simulink model "HeartCode"  (R2020a)
settings: Solver=FixedStepAuto  StartTime=0.0  StopTime=10.0  FixedStep=1e-3  RelTol=1e-3  EnableMultiTasking=on
undefined symbols (not defined in the file): A0, A1, D0, D1, D10, D11, D12, D13, D2, D3, D4, D5, D6, D7, D8, D9, PTA0, PTA1, PTA2, PTB2, PTB23, PTB3, PTB9, PTC16, PTC17, PTC2, PTC3, PTC4, PTD0, PTD1, PTD2, PTD3
libraries: frdmk64flib x21, etargetslib x10
settings Model: ExtModeTrigDuration=5  Creator=user  LastModifiedBy=user
settings OptimizationCC: EnhancedBackFolding=on  PassReuseOutputArgsAs=Individual arguments  ZeroExternalMemoryAtStartup=off  ZeroInternalMemoryAtStartup=off  MaxStackSize=64  OptimizeBlockOrder=speed  DifferentSizesBufferReuse=on  OptimizationCustomize=off  EfficientTunableParamExpr=on
settings DebuggingCC: ParameterTunabilityLossMsg=error
settings HardwareCC: ProdBitPerPointer=32  ProdBitPerSizeT=32  ProdBitPerPtrDiffT=32  ProdLargestAtomicInteger=Long  ProdLargestAtomicFloat=Double  ProdWordSize=32  ProdHWDeviceType=ARM Compatible->ARM Cortex
settings SFSimCC: MATLABDynamicMemAlloc=off
settings RTWCC: SystemTargetFile=ert.tlc  HardwareBoard=NXP FRDM-K64F  TemplateMakefile=ert_default_tmf  Toolchain=GNU Tools for ARM Embedded Processors
settings CodeAppCC: ForceParamTrailComments=on  IgnoreCustomStorageClasses=off  OperatorAnnotations=on  SimulinkDataObjDesc=on  SFDataObjDesc=on  InsertBlockDesc=on

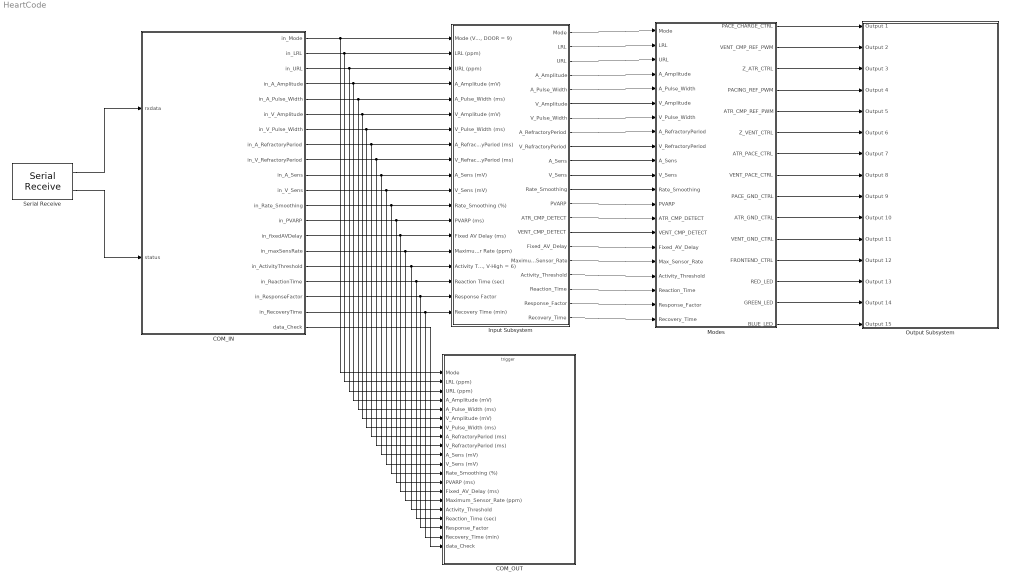
== system HeartCode ==
  COM_IN : Stateflow chart  TreatAsAtomicUnit=on
  COM_OUT : Subsystem  TreatAsAtomicUnit=on
  Input Subsystem : Subsystem
  Modes : Stateflow chart  TreatAsAtomicUnit=on
  Output Subsystem : Subsystem
  Serial Receive : frdmk64flib/Serial Receive  SCIModule=0  Baudrate=uint32(9600)  Parity=None  StopBits=1  HardwareFlowControl=None  ByteOrder=LittleEndian  DataType=uint8  DataLength=33  BlockingMode=off  OutputStatus=on  SampleTime=-1
  wires:
  Modes/1(PACE_CHARGE_CTRL) -> Output Subsystem/1(Output 1)
  Modes/2(VENT_CMP_REF_PWM) -> Output Subsystem/2(Output 2)
  Modes/3(Z_ATR_CTRL) -> Output Subsystem/3(Output 3)
  Modes/4(PACING_REF_PWM) -> Output Subsystem/4(Output 4)
  Modes/5(ATR_CMP_REF_PWM) -> Output Subsystem/5(Output 5)
  Modes/6(Z_VENT_CTRL) -> Output Subsystem/6(Output 6)
  Modes/7(ATR_PACE_CTRL) -> Output Subsystem/7(Output 7)
  Modes/8(VENT_PACE_CTRL) -> Output Subsystem/8(Output 8)
  Modes/9(PACE_GND_CTRL) -> Output Subsystem/9(Output 9)
  Modes/10(ATR_GND_CTRL) -> Output Subsystem/10(Output 10)
  Modes/11(VENT_GND_CTRL) -> Output Subsystem/11(Output 11)
  Modes/12(FRONTEND_CTRL) -> Output Subsystem/12(Output 12)
  Modes/13(RED_LED) -> Output Subsystem/13(Output 13)
  Modes/14(GREEN_LED) -> Output Subsystem/14(Output 14)
  Modes/15(BLUE_LED) -> Output Subsystem/15(Output 15)
  Input Subsystem/2(LRL) -> Modes/2(LRL)
  Input Subsystem/3(URL) -> Modes/3(URL)
  Input Subsystem/4(A_Amplitude) -> Modes/4(A_Amplitude)
  Input Subsystem/5(A_Pulse_Width) -> Modes/5(A_Pulse_Width)
  Input Subsystem/6(V_Amplitude) -> Modes/6(V_Amplitude)
  Input Subsystem/7(V_Pulse_Width) -> Modes/7(V_Pulse_Width)
  Input Subsystem/10(A_Sens) -> Modes/10(A_Sens)
  Input Subsystem/11(V_Sens) -> Modes/11(V_Sens)
  Input Subsystem/12(Rate_Smoothing) -> Modes/12(Rate_Smoothing)
  Input Subsystem/13(PVARP) -> Modes/13(PVARP)
  Input Subsystem/1(Mode) -> Modes/1(Mode)
  Input Subsystem/14(ATR_CMP_DETECT) -> Modes/14(ATR_CMP_DETECT)
  Input Subsystem/15(VENT_CMP_DETECT) -> Modes/15(VENT_CMP_DETECT)
  Input Subsystem/8(A_RefractoryPeriod) -> Modes/8(A_RefractoryPeriod)
  Input Subsystem/9(V_RefractoryPeriod) -> Modes/9(V_RefractoryPeriod)
  Input Subsystem/16(Fixed_AV_Delay) -> Modes/16(Fixed_AV_Delay)
  Input Subsystem/17(Maximum_Sensor_Rate) -> Modes/17(Max_Sensor_Rate)
  Input Subsystem/18(Activity_Threshold) -> Modes/18(Activity_Threshold)
  Input Subsystem/19(Reaction_Time) -> Modes/19(Reaction_Time)
  Input Subsystem/20(Response_Factor) -> Modes/20(Response_Factor)
  Input Subsystem/21(Recovery_Time) -> Modes/21(Recovery_Time)
  Serial Receive/1 -> COM_IN/1(rxdata)
  Serial Receive/2 -> COM_IN/2(status)
  COM_IN/1(in_Mode) -> Input Subsystem/1("Mode (VOO = 0, VVI = 1, AOO = 2, AAI = 3, DOO = 4) (VOOR = 5, VVIR = 6, AOOR = 7, AAIR = 8, DOOR = 9)"), COM_OUT/1(Mode)
  COM_IN/2(in_LRL) -> Input Subsystem/2(LRL (ppm)), COM_OUT/2(LRL (ppm))
  COM_IN/3(in_URL) -> Input Subsystem/3(URL (ppm)), COM_OUT/3(URL (ppm))
  COM_IN/4(in_A_Amplitude) -> Input Subsystem/4(A_Amplitude (mV)), COM_OUT/4(A_Amplitude (mV))
  COM_IN/5(in_A_Pulse_Width) -> Input Subsystem/5(A_Pulse_Width (ms)), COM_OUT/5(A_Pulse_Width (ms))
  COM_IN/6(in_V_Amplitude) -> Input Subsystem/6(V_Amplitude (mV)), COM_OUT/6(V_Amplitude (mV))
  COM_IN/7(in_V_Pulse_Width) -> Input Subsystem/7(V_Pulse_Width (ms)), COM_OUT/7(V_Pulse_Width (ms))
  COM_IN/8(in_A_RefractoryPeriod) -> Input Subsystem/8(A_RefractoryPeriod (ms)), COM_OUT/8(A_RefractoryPeriod (ms))
  COM_IN/9(in_V_RefractoryPeriod) -> Input Subsystem/9(V_RefractoryPeriod (ms)), COM_OUT/9(V_RefractoryPeriod (ms))
  COM_IN/11(in_V_Sens) -> Input Subsystem/11(V_Sens (mV)), COM_OUT/11(V_Sens (mV))
  COM_IN/12(in_Rate_Smoothing) -> Input Subsystem/12(Rate_Smoothing (%)), COM_OUT/12(Rate_Smoothing (%))
  COM_IN/13(in_PVARP) -> Input Subsystem/13(PVARP (ms)), COM_OUT/13(PVARP (ms))
  COM_IN/14(in_fixedAVDelay) -> Input Subsystem/14(Fixed AV Delay (ms)), COM_OUT/14(Fixed_AV_Delay (ms))
  COM_IN/16(in_ActivityThreshold) -> Input Subsystem/16("Activity Threshold (V-Low = 0, Low = 1, Med-Low = 2, Med = 3) (Med-High = 4, High = 5, V-High = 6)"), COM_OUT/16(Activity_Threshold)
  COM_IN/17(in_ReactionTime) -> Input Subsystem/17(Reaction Time (sec)), COM_OUT/17(Reaction_Time (sec))
  COM_IN/18(in_ResponseFactor) -> Input Subsystem/18(Response Factor), COM_OUT/18(Response_Factor)
  COM_IN/19(in_RecoveryTime) -> Input Subsystem/19(Recovery Time (min)), COM_OUT/19(Recovery_Time (min))
  COM_IN/10(in_A_Sens) -> Input Subsystem/10(A_Sens (mV)), COM_OUT/10(A_Sens (mV))
  COM_IN/15(in_maxSensRate) -> Input Subsystem/15(Maximum Sensor Rate (ppm)), COM_OUT/15(Maximum_Sensor_Rate (ppm))
  COM_IN/20(data_Check) -> COM_OUT/20(data_Check)

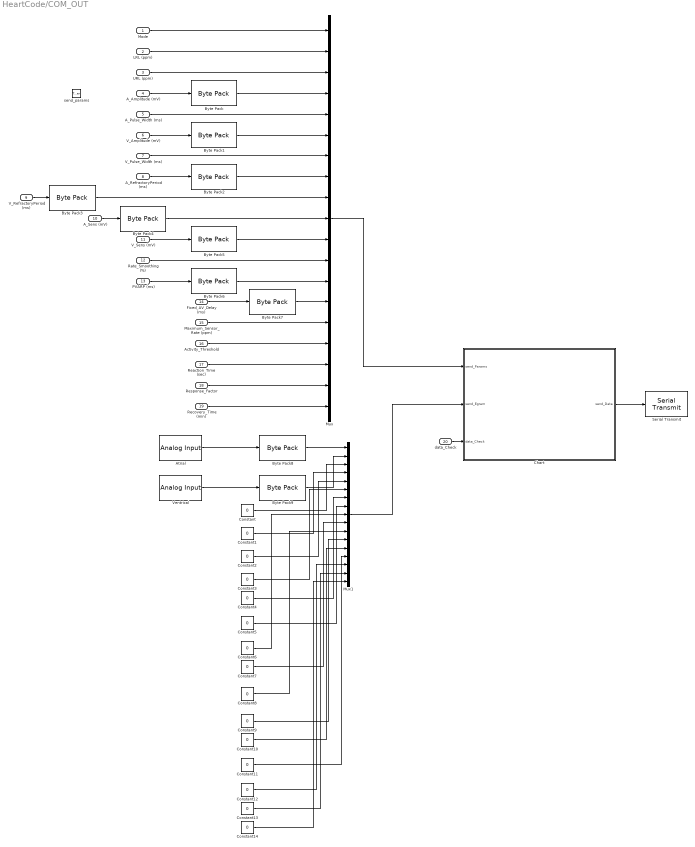
== system HeartCode/COM_OUT ==
  Mode : Inport
  LRL (ppm) : Inport  Port=2
  URL (ppm) : Inport  Port=3
  A_Amplitude (mV) : Inport  Port=4
  A_Pulse_Width (ms) : Inport  Port=5
  V_Amplitude (mV) : Inport  Port=6
  V_Pulse_Width (ms) : Inport  Port=7
  A_RefractoryPeriod (ms) : Inport  Port=8
  V_RefractoryPeriod (ms) : Inport  Port=9
  A_Sens (mV) : Inport  Port=10
  V_Sens (mV) : Inport  Port=11
  Rate_Smoothing (%) : Inport  Port=12
  PVARP (ms) : Inport  Port=13
  Fixed_AV_Delay (ms) : Inport  Port=14
  Maximum_Sensor_Rate (ppm) : Inport  Port=15
  Activity_Threshold : Inport  Port=16
  Reaction_Time (sec) : Inport  Port=17
  Response_Factor : Inport  Port=18
  Recovery_Time (min) : Inport  Port=19
  data_Check : Inport  Port=20
  send_params : TriggerPort  TriggerType=function-call  IsSimulinkFunction=on  FunctionName=send_params  VariantControl=Variant
  Atrial : frdmk64flib/Analog Input  Whichpin=PTB2 (A0)  SampleTime=-1
  Byte Pack{,1..3,6..7} (6 alike) : etargetslib/Byte Pack  datatypes={'uint16'}  byteAlign=1
  Byte Pack4 : etargetslib/Byte Pack  datatypes={'single'}  byteAlign=1
  Byte Pack5 : etargetslib/Byte Pack  datatypes={'single'}  byteAlign=1
  Byte Pack8 : etargetslib/Byte Pack  datatypes={'double'}  byteAlign=1
  Byte Pack9 : etargetslib/Byte Pack  datatypes={'double'}  byteAlign=1
  Chart : Stateflow chart  TreatAsAtomicUnit=on
  Constant{,1..14} (15 alike) : Constant  Value=0  OutDataTypeStr=uint8
  Mux : Mux  Inputs=19
  Mux1 : Mux  Inputs=17
  Serial Transmit : frdmk64flib/Serial Transmit  SCIModule=0  Baudrate=uint32(9600)  Parity=None  StopBits=1  HardwareFlowControl=None  ByteOrder=LittleEndian  BlockingMode=on  OutputStatus=off
  Ventrical : frdmk64flib/Analog Input  Whichpin=PTB3 (A1)  SampleTime=-1
  wires:
  LRL (ppm)/1 -> Mux/2
  Mux/1 -> Chart/1(send_Params)
  URL (ppm)/1 -> Mux/3
  A_Amplitude (mV)/1 -> Byte Pack/1
  A_Pulse_Width (ms)/1 -> Mux/5
  V_Amplitude (mV)/1 -> Byte Pack1/1
  V_Pulse_Width (ms)/1 -> Mux/7
  A_RefractoryPeriod (ms)/1 -> Byte Pack2/1
  V_RefractoryPeriod (ms)/1 -> Byte Pack3/1
  A_Sens (mV)/1 -> Byte Pack4/1
  V_Sens (mV)/1 -> Byte Pack5/1
  Rate_Smoothing (%)/1 -> Mux/12
  PVARP (ms)/1 -> Byte Pack6/1
  Mode/1 -> Mux/1
  Fixed_AV_Delay (ms)/1 -> Byte Pack7/1
  Maximum_Sensor_Rate (ppm)/1 -> Mux/15
  Reaction_Time (sec)/1 -> Mux/17
  Response_Factor/1 -> Mux/18
  Recovery_Time (min)/1 -> Mux/19
  Byte Pack/1 -> Mux/4
  Byte Pack1/1 -> Mux/6
  Byte Pack2/1 -> Mux/8
  Byte Pack3/1 -> Mux/9
  Byte Pack4/1 -> Mux/10
  Byte Pack5/1 -> Mux/11
  Byte Pack6/1 -> Mux/13
  Byte Pack7/1 -> Mux/14
  Activity_Threshold/1 -> Mux/16
  data_Check/1 -> Chart/3(data_Check)
  Chart/1(send_Data) -> Serial Transmit/1
  Atrial/1 -> Byte Pack8/1
  Ventrical/1 -> Byte Pack9/1
  Constant1/1 -> Mux1/4
  Constant2/1 -> Mux1/5
  Constant14/1 -> Mux1/17
  Constant13/1 -> Mux1/16
  Constant12/1 -> Mux1/15
  Constant11/1 -> Mux1/14
  Constant10/1 -> Mux1/13
  Constant9/1 -> Mux1/12
  Constant8/1 -> Mux1/11
  Constant7/1 -> Mux1/10
  Constant6/1 -> Mux1/9
  Constant5/1 -> Mux1/8
  Constant4/1 -> Mux1/7
  Constant3/1 -> Mux1/6
  Byte Pack8/1 -> Mux1/1
  Byte Pack9/1 -> Mux1/2
  Constant/1 -> Mux1/3
  Mux1/1 -> Chart/2(send_Egram)

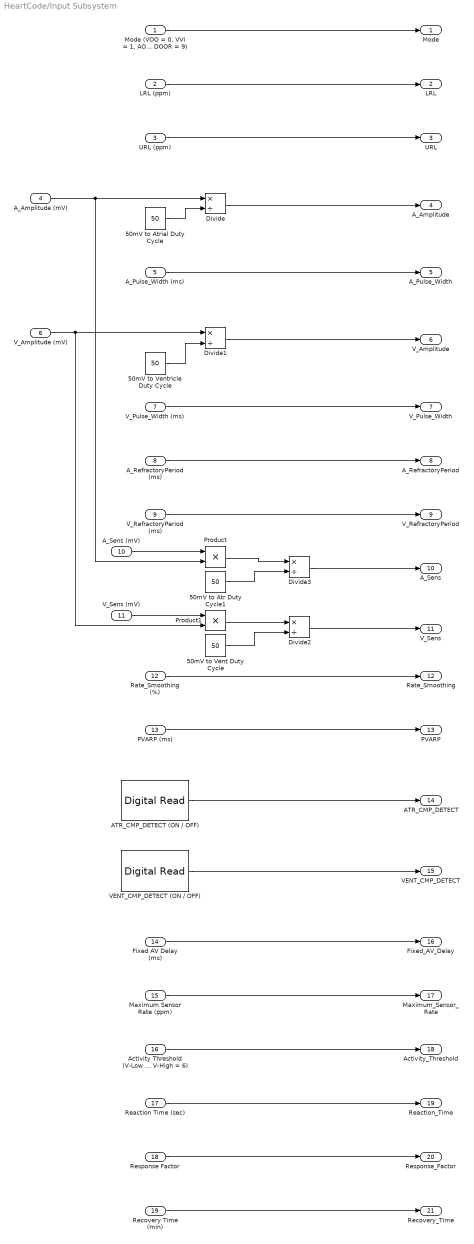
== system HeartCode/Input Subsystem ==
  "Mode (VOO = 0, VVI = 1, AOO = 2, AAI = 3, DOO = 4) (VOOR = 5, VVIR = 6, AOOR = 7, AAIR = 8, DOOR = 9)" : Inport
  LRL (ppm) : Inport  Port=2
  URL (ppm) : Inport  Port=3
  A_Amplitude (mV) : Inport  Port=4
  A_Pulse_Width (ms) : Inport  Port=5
  V_Amplitude (mV) : Inport  Port=6
  V_Pulse_Width (ms) : Inport  Port=7
  A_RefractoryPeriod (ms) : Inport  Port=8
  V_RefractoryPeriod (ms) : Inport  Port=9
  A_Sens (mV) : Inport  Port=10
  V_Sens (mV) : Inport  Port=11
  Rate_Smoothing (%) : Inport  Port=12
  PVARP (ms) : Inport  Port=13
  Fixed AV Delay (ms) : Inport  Port=14
  Maximum Sensor Rate (ppm) : Inport  Port=15
  "Activity Threshold (V-Low = 0, Low = 1, Med-Low = 2, Med = 3) (Med-High = 4, High = 5, V-High = 6)" : Inport  Port=16
  Reaction Time (sec) : Inport  Port=17
  Response Factor : Inport  Port=18
  Recovery Time (min) : Inport  Port=19
  50mV to Atr Duty Cycle1 : Constant  Value=50
  50mV to Atrial Duty Cycle : Constant  Value=50
  50mV to Vent Duty Cycle : Constant  Value=50
  50mV to Ventricle Duty Cycle : Constant  Value=50
  ATR_CMP_DETECT (ON / OFF) : frdmk64flib/Digital Read  Whichpin=PTC16 (D0)  SampleTime=-1
  Divide{,1..3} (4 alike) : Product  Inputs=*/
  Product : Product
  Product1 : Product
  VENT_CMP_DETECT (ON / OFF) : frdmk64flib/Digital Read  Whichpin=PTC17 (D1)  SampleTime=-1
  Mode : Outport
  LRL : Outport  Port=2
  URL : Outport  Port=3
  A_Amplitude : Outport  Port=4
  A_Pulse_Width : Outport  Port=5
  V_Amplitude : Outport  Port=6
  V_Pulse_Width : Outport  Port=7
  A_RefractoryPeriod : Outport  Port=8
  V_RefractoryPeriod : Outport  Port=9
  A_Sens : Outport  Port=10
  V_Sens : Outport  Port=11
  Rate_Smoothing : Outport  Port=12
  PVARP : Outport  Port=13
  ATR_CMP_DETECT : Outport  Port=14
  VENT_CMP_DETECT : Outport  Port=15
  Fixed_AV_Delay : Outport  Port=16
  Maximum_Sensor_Rate : Outport  Port=17
  Activity_Threshold : Outport  Port=18
  Reaction_Time : Outport  Port=19
  Response_Factor : Outport  Port=20
  Recovery_Time : Outport  Port=21
  wires:
  V_RefractoryPeriod (ms)/1 -> V_RefractoryPeriod/1
  URL (ppm)/1 -> URL/1
  VENT_CMP_DETECT (ON / OFF)/1 -> VENT_CMP_DETECT/1
  V_Pulse_Width (ms)/1 -> V_Pulse_Width/1
  "Mode (VOO = 0, VVI = 1, AOO = 2, AAI = 3, DOO = 4) (VOOR = 5, VVIR = 6, AOOR = 7, AAIR = 8, DOOR = 9)"/1 -> Mode/1
  ATR_CMP_DETECT (ON / OFF)/1 -> ATR_CMP_DETECT/1
  A_Pulse_Width (ms)/1 -> A_Pulse_Width/1
  PVARP (ms)/1 -> PVARP/1
  LRL (ppm)/1 -> LRL/1
  A_RefractoryPeriod (ms)/1 -> A_RefractoryPeriod/1
  Rate_Smoothing (%)/1 -> Rate_Smoothing/1
  A_Amplitude (mV)/1 -> Divide/1, Product/2
  50mV to Atrial Duty Cycle/1 -> Divide/2
  Divide/1 -> A_Amplitude/1
  V_Amplitude (mV)/1 -> Divide1/1, Product1/2
  50mV to Ventricle Duty Cycle/1 -> Divide1/2
  Divide1/1 -> V_Amplitude/1
  A_Sens (mV)/1 -> Product/1
  V_Sens (mV)/1 -> Product1/1
  Product1/1 -> Divide2/1
  50mV to Vent Duty Cycle/1 -> Divide2/2
  Divide2/1 -> V_Sens/1
  Product/1 -> Divide3/1
  50mV to Atr Duty Cycle1/1 -> Divide3/2
  Divide3/1 -> A_Sens/1
  Fixed AV Delay (ms)/1 -> Fixed_AV_Delay/1
  Maximum Sensor Rate (ppm)/1 -> Maximum_Sensor_Rate/1
  "Activity Threshold (V-Low = 0, Low = 1, Med-Low = 2, Med = 3) (Med-High = 4, High = 5, V-High = 6)"/1 -> Activity_Threshold/1
  Reaction Time (sec)/1 -> Reaction_Time/1
  Response Factor/1 -> Response_Factor/1
  Recovery Time (min)/1 -> Recovery_Time/1

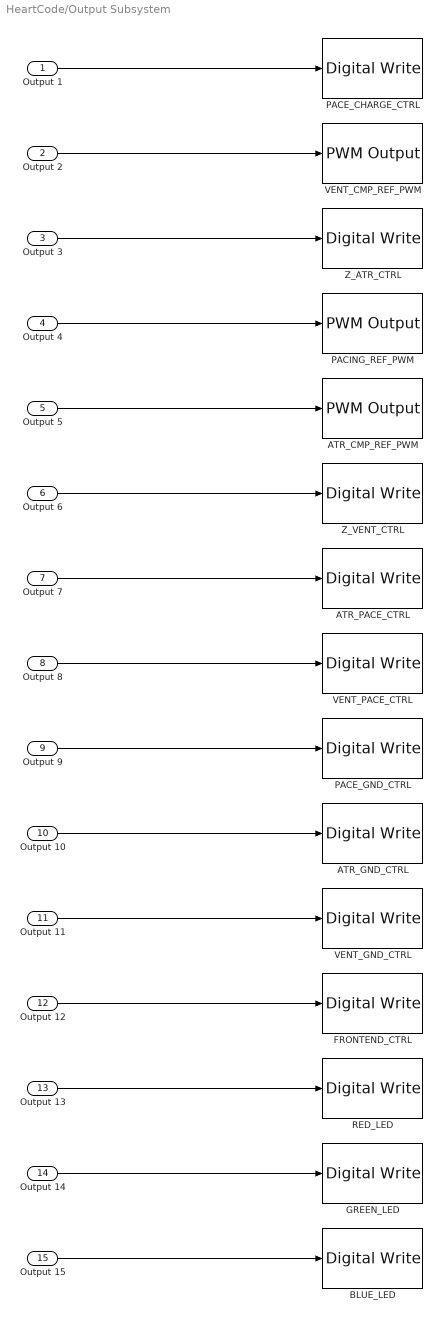
== system HeartCode/Output Subsystem ==
  Output 1 : Inport
  Output 2 : Inport  Port=2
  Output 3 : Inport  Port=3
  Output 4 : Inport  Port=4
  Output 5 : Inport  Port=5
  Output 6 : Inport  Port=6
  Output 7 : Inport  Port=7
  Output 8 : Inport  Port=8
  Output 9 : Inport  Port=9
  Output 10 : Inport  Port=10
  Output 11 : Inport  Port=11
  Output 12 : Inport  Port=12
  Output 13 : Inport  Port=13
  Output 14 : Inport  Port=14
  Output 15 : Inport  Port=15
  ATR_CMP_REF_PWM : frdmk64flib/PWM Output  Whichpin=PTC2 (D6)  InitialFrequency=2000  InitialDutyCycle=100
  ATR_GND_CTRL : frdmk64flib/Digital Write  Whichpin=PTD2 (D11)
  ATR_PACE_CTRL : frdmk64flib/Digital Write  Whichpin=PTA0 (D8)
  BLUE_LED : frdmk64flib/Digital Write  Whichpin=BLUE_LED
  FRONTEND_CTRL : frdmk64flib/Digital Write  Whichpin=PTD1 (D13)
  GREEN_LED : frdmk64flib/Digital Write  Whichpin=GREEN_LED
  PACE_CHARGE_CTRL : frdmk64flib/Digital Write  Whichpin=PTB9 (D2)
  PACE_GND_CTRL : frdmk64flib/Digital Write  Whichpin=PTD0 (D10)
  PACING_REF_PWM : frdmk64flib/PWM Output  Whichpin=PTA2 (D5)  InitialFrequency=2000  InitialDutyCycle=100
  RED_LED : frdmk64flib/Digital Write  Whichpin=RED_LED
  VENT_CMP_REF_PWM : frdmk64flib/PWM Output  Whichpin=PTA1 (D3)  InitialFrequency=2000  InitialDutyCycle=100
  VENT_GND_CTRL : frdmk64flib/Digital Write  Whichpin=PTD3 (D12)
  VENT_PACE_CTRL : frdmk64flib/Digital Write  Whichpin=PTC4 (D9)
  Z_ATR_CTRL : frdmk64flib/Digital Write  Whichpin=PTB23 (D4)
  Z_VENT_CTRL : frdmk64flib/Digital Write  Whichpin=PTC3 (D7)
  wires:
  Output 11/1 -> VENT_GND_CTRL/1
  Output 1/1 -> PACE_CHARGE_CTRL/1
  Output 10/1 -> ATR_GND_CTRL/1
  Output 15/1 -> BLUE_LED/1
  Output 3/1 -> Z_ATR_CTRL/1
  Output 13/1 -> RED_LED/1
  Output 6/1 -> Z_VENT_CTRL/1
  Output 9/1 -> PACE_GND_CTRL/1
  Output 8/1 -> VENT_PACE_CTRL/1
  Output 4/1 -> PACING_REF_PWM/1
  Output 5/1 -> ATR_CMP_REF_PWM/1
  Output 7/1 -> ATR_PACE_CTRL/1
  Output 2/1 -> VENT_CMP_REF_PWM/1
  Output 12/1 -> FRONTEND_CTRL/1
  Output 14/1 -> GREEN_LED/1

== stateflow chart HeartCode/COM_IN ==
  settings: executeAtInitialization=1
  state SET_PARAM
    entry:
    in_Mode = rxdata(3);
    in_LRL = rxdata(4);
    in_URL = rxdata(5);
    in_A_Amplitude = typecast(rxdata(6:7),'uint16');
    in_A_Pulse_Width = rxdata(8);
    in_V_Amplitude = typecast(rxdata(9:10),'uint16');
    in_V_Pulse_Width = rxdata(11);
    in_A_RefractoryPeriod = typecast(rxdata(12:13),'uint16');
    in_V_RefractoryPeriod = typecast(rxdata(14:15),'uint16');
    in_A_Sens = typecast(rxdata(16:19),'single');
    in_V_Sens = typecast(rxdata(20:23),'single');
    in_Rate_Smoothing = rxdata(24);
    in_PVARP = typecast(rxdata(25:26),'uint16');
    in_fixedAVDelay = typecast(rxdata(27:28),'uint16');
    in_maxSensRate  = rxdata(29);
    in_ActivityThreshold = rxdata(30);
    in_ReactionTime = rxdata(31);
    in_ResponseFactor = rxdata(32);
    in_RecoveryTime = rxdata(33);
  state INITIAL
    %Set the initial values of parameters
    entry:
    in_Mode = 0;
    in_LRL = 120;
    in_URL = 130;
    in_A_Amplitude = 4000;
    in_A_Pulse_Width = 10;
    in_V_Amplitude = 3500;
    in_V_Pulse_Width = 10;
    in_A_RefractoryPeriod = 100;
    in_V_RefractoryPeriod = 100;
    in_A_Sens = 0.75;
    in_V_Sens = 1.0;
    in_Rate_Smoothing = 0;
    in_PVARP = 250;
    in_fixedAVDelay = 150;
    in_maxSensRate = 120;
    in_ActivityThreshold = 3;
    in_ReactionTime = 30;
    in_ResponseFactor = 8;
    in_RecoveryTime = 5;
  state STANDBY
    %Waiting for COM
  state ECHO_PARAM
    entry:
    data_Check = rxdata(2);
    send_params();
  state ECHO_EGRAM
    entry:
    data_Check = rxdata(2);
    send_params();
  (default) -> INITIAL
  SET_PARAM -> STANDBY
  (junction 9) -> SET_PARAM [order 2] : [rxdata(2) == hex2dec('55')]
  (junction 7) -> STANDBY [order 2]
  (junction 9) -> ECHO_EGRAM [order 3] : [rxdata(2) == hex2dec('47')]
  INITIAL -> STANDBY
  STANDBY -> (junction 7) : [status == 0]
  (junction 7) -> (junction 9) [order 1] : [rxdata(1) == hex2dec('16')]
  (junction 9) -> ECHO_PARAM [order 1] : [rxdata(2) == hex2dec('22')]
  ECHO_EGRAM -> STANDBY [order 2] : [rxdata(2) == hex2dec('62')]
  ECHO_PARAM -> STANDBY
  ECHO_EGRAM -> ECHO_EGRAM [order 1] : [after(100, msec)]
  data: in_Mode output uint8; rxdata input uint8; status input uint8; in_LRL output uint8; in_URL output uint8; in_A_Amplitude output uint16; in_A_Pulse_Width output uint8; in_V_Amplitude output uint16; in_V_Pulse_Width output uint8; in_A_RefractoryPeriod output uint16; in_V_RefractoryPeriod output uint16; in_A_Sens output single; in_V_Sens output single; in_Rate_Smoothing output uint8; in_PVARP output uint16; in_fixedAVDelay output uint16; in_maxSensRate output uint8; in_ActivityThreshold output uint8; in_ReactionTime output uint8; in_ResponseFactor output uint8; in_RecoveryTime output uint8; data_Check output uint8

== stateflow chart HeartCode/COM_OUT/Chart ==
  state SEND_PARAMETERS
    entry:
    send_Data = send_Params;
  state INITIAL
  state SEND_EGRAM
    entry:
    send_Data = send_Egram;
  SEND_PARAMETERS -> INITIAL
  INITIAL -> SEND_PARAMETERS [order 2] : [data_Check == hex2dec('22')]
  (default) -> INITIAL
  SEND_EGRAM -> INITIAL
  INITIAL -> SEND_EGRAM [order 1] : [data_Check == hex2dec('47')]
  data: send_Params input uint8; send_Egram input uint8; data_Check input uint8; send_Data output uint8 size=31

== stateflow chart HeartCode/Modes ==
  note: Since in the main state, FRONTEND_CTRL is true so the
      | microcontroller enables sensing. The pacemaker then waits
      | until after the ventricle refractory period (V_RefractoryPeriod)
      | and if the current mode is set to VVI (Mode 1) and the
      | microcontroller senses a natural pace in the ventricle
      | (VENT_CMP_DETECT is true), it loops back into VOO_Charging
      | to inhibit the next ventricle pace. The microcontroller registers a
      | pace when the ventricle threshold sensitivity is exceeded which
      | is represented by the value of V_Sens stored into
      | VENT_CMP_REF_PWM. After using the MCP6546 Comparator
      | within the microcontroller to compare the rectified signal and
      | the PWM threshold, the output would trigger a response through
      | the VENT_CMP_DETECT pin which indicates that the ventricle
      | triggered a pulse.
  state VVI
    %To show when Ventricular pace being inhibited
    entry:
    RED_LED = true;
  state VOO_Charging
    %Charging C22 and Discharging Blocking Capacitor
    entry:
    ATR_PACE_CTRL = false;
    VENT_PACE_CTRL = false;
    PACING_REF_PWM = V_Amplitude;
    PACE_CHARGE_CTRL = true;
    %Discharging Blocking Capacitor
    PACE_GND_CTRL = true;
    Z_ATR_CTRL = false;
    Z_VENT_CTRL = false;
    ATR_GND_CTRL = false;
    VENT_GND_CTRL = true;
    GREEN_LED = false;
    %Needed for VENT_CMP_DETECT
    VENT_CMP_REF_PWM = V_Sens;
  state VOO_Pacing
    %Discharging C22
    entry:
    PACE_CHARGE_CTRL = false;
    PACE_GND_CTRL = true;
    ATR_PACE_CTRL = false;
    ATR_GND_CTRL = false;
    Z_ATR_CTRL = false;
    Z_VENT_CTRL = false;
    VENT_GND_CTRL = false;
    VENT_PACE_CTRL = true;
    GREEN_LED = true;
  note: Move from ventricle pacing state back to charging
      | the C22 capacitor after the programmed ventricle
      | pulse width.
  note: The state becomes ready for pacing after a delay
      | which is indicated by the time interval between
      | the ventricle paces. This time interval is represented
      | by 60000 divided by the lower rate limit in ppm
      | subtracted by the programmed ventricular pulse width.
  note: If the mode is set to VOO or VVI,
      | proceed to the next state
  note: In the charging state, the C22 capacitor is charged and the blocking
      | capacitor is discharged. To charge the C22 capacitor,
      | PACE_CHARGE_CTRL is set to true to charge the pacing capacitor,
      | and both ATR_PACE_CTRL and VENT_PACE_CTRL is set to false
      | to prevent the patient from being directly connected to the input
      | charging signal. To simultaneously discharge the blocking capacitor,
      | the net charge build-up in the ventricle/atrium must be reduced to
      | zero. For the specific mode, the GND_CTRL is set to true to act as
      | a pull-down for the electrode in order to prevent unwanted pacing.
      | The GND_CTRL for the other mode is set to false along with the
      | Z_ATR_CTRL and Z_VENT_CTRL so there is no impedance in the
      | respective chambers.
  note: In the pacing state, the charged C22 capacitor applies a pace to
      | either the ventricle or atirum depending on the mode. The power
      | supply is cut off the circuit by setting PACE_CHARGE_CTRL
      | to false and the switch PACE_CTRL is turned on to direct current
      | towards the specific chamber for the current mode. Only the specific
      | pacing switch for the current mode is true while the other is made
      | false to prevent parallel connection. The GND_CTRL for both atrial
      | and ventricular are turned false to ensure that the pacing signals
      | do not flow back into ground. Z_ATR_CTRL and Z_VENT_CTRL
      | remains false so that there is no impedance within the atrial and
      | ventricular chambers.
  note: The state becomes ready for pacing after a delay
      | which is indicated by the time interval between
      | the atrial paces. This time interval is represented
      | by 60000 divided by the lower rate limit in ppm
      | subtracted by the programmed atrial pulse width.
  state AOO_Charging
    %Charging C22 and Discharging Blocking Capacitor
    entry:
    ATR_PACE_CTRL = false;
    VENT_PACE_CTRL = false;
    PACING_REF_PWM = A_Amplitude;
    PACE_CHARGE_CTRL = true;
    %Discharging Blocking Capacitor
    PACE_GND_CTRL = true;
    Z_ATR_CTRL = false;
    Z_VENT_CTRL = false;
    ATR_GND_CTRL = true;
    VENT_GND_CTRL = false;
    BLUE_LED=false;
    RED_LED = false;
    %Needed for ATR_CMP_DETECT
    ATR_CMP_REF_PWM = A_Sens;
  state AOO_Pacing
    %Discharging C22
    entry:
    PACE_CHARGE_CTRL = false;
    PACE_GND_CTRL = true;
    ATR_PACE_CTRL = true;
    ATR_GND_CTRL = false;
    Z_ATR_CTRL = false;
    Z_VENT_CTRL = false;
    VENT_GND_CTRL = false;
    VENT_PACE_CTRL = false;
    BLUE_LED = true;
  state Main
    entry:
    BLUE_LED = false;
    RED_LED = false;
    GREEN_LED = false;
    PACING_REF_PWM = 0;
    FRONTEND_CTRL = true;
  note: Move from atrial pacing state back to charging
      | the C22 capacitor after the programmed atrial
      | pulse width.
  note: If the mode is set to AOO or AAI,
      | proceed to the next state
  note: In the main state, all LED indicators are
      | initialized to false. The variable
      | FRONTEND_CTRL is initialized to true in
      | order to activate sensing. There are two
      |  transitions to the other states based on
      | the mode that was selected.
  state AAI
    %To show when Atrial pace being inhibited
    entry:
    RED_LED = true;
  note: Since in the main state, FRONTEND_CTRL is true so the
      | microcontroller enables sensing. The pacemaker then waits
      | until after the atrial refractory period (A_RefractoryPeriod)
      | and if the current mode is set to AAI (Mode 3) and the
      | microcontroller senses a natural pace in the atrium
      | (ATR_CMP_DETECT is true), it loops back into AOO_Charging
      | to inhibit the next atrium pace. The microcontroller registers a
      | pace when the atrium threshold sensitivity is exceeded which
      | is represented by the value of A_Sens stored into
      | ATR_CMP_REF_PWM. After using the MCP6546 Comparator
      | within the microcontroller to compare the rectified signal and
      | the PWM threshold, the output would trigger a response through
      | the ATR_CMP_DETECT pin which indicates that the atrium triggered
      | a pulse.
  note: If the mode is set to DOO,
      | proceed to the next state
  state DOO_Charging
    %Charging C22 and Discharging Blocking Capacitor
    entry:
    %AOO_Charging
    ATR_PACE_CTRL = false;
    VENT_PACE_CTRL = false;
    PACING_REF_PWM = A_Amplitude;
    PACE_CHARGE_CTRL = true;
    %Discharging Blocking Capacitor for Ventricle
    PACE_GND_CTRL = true;
    Z_ATR_CTRL = false;
    Z_VENT_CTRL = false;
    ATR_GND_CTRL = false;
    VENT_GND_CTRL = true;
    BLUE_LED=false;
    GREEN_LED = false;
  state DOO_Pacing
    %Discharging C22
    entry:
    %AOO_Pacing
    PACE_CHARGE_CTRL = false;
    PACE_GND_CTRL = true;
    ATR_PACE_CTRL = true;
    ATR_GND_CTRL = false;
    Z_ATR_CTRL = false;
    Z_VENT_CTRL = false;
    VENT_GND_CTRL = false;
    VENT_PACE_CTRL = false;
    BLUE_LED = true;
  state DOO_Charging1
    %Charging C22 and Discharging Blocking Capacitor
    entry:
    %VOO_Charging
    ATR_PACE_CTRL = false;
    VENT_PACE_CTRL = false;
    PACING_REF_PWM = V_Amplitude;
    PACE_CHARGE_CTRL = true;
    %Discharging Blocking Capacitor for Atrium
    PACE_GND_CTRL = true;
    Z_ATR_CTRL = false;
    Z_VENT_CTRL = false;
    ATR_GND_CTRL = true;
    VENT_GND_CTRL = false;
    BLUE_LED = false;
    GREEN_LED = false;
  state DOO_Pacing1
    %Discharging C22
    entry:
    %VOO_Pacing
    PACE_CHARGE_CTRL = false;
    PACE_GND_CTRL = true;
    ATR_PACE_CTRL = false;
    ATR_GND_CTRL = false;
    Z_ATR_CTRL = false;
    Z_VENT_CTRL = false;
    VENT_GND_CTRL = false;
    VENT_PACE_CTRL = true;
    GREEN_LED = true;
  (junction 122) -> VVI [order 2] : [Mode == 1]
  VOO_Charging -> VVI [order 2] : [Mode == 1 && VENT_CMP_DETECT == true]{VdeltaT = 0}
  VVI -> VOO_Charging : after(V_RefractoryPeriod, msec){VdeltaT = VdeltaT + V_RefractoryPeriod}
  (junction 122) -> VOO_Charging [order 1] : [Mode==0]
  VOO_Pacing -> (junction 122) : after(V_Pulse_Width,msec){VdeltaT = VdeltaT + uint16(V_Pulse_Width)}
  Main -> VOO_Charging [order 2] : [Mode == 0 || Mode == 1]
  VOO_Charging -> VOO_Pacing [order 1] : after([60000/uint16(LRL)] - VdeltaT, msec){VdeltaT = 0}
  (default) -> Main
  AOO_Charging -> AOO_Pacing [order 1] : after((60000/uint16(LRL)) - AdeltaT, msec){AdeltaT = 0}
  Main -> AOO_Charging [order 1] : [Mode==2 || Mode == 3]
  Main -> DOO_Charging [order 3] : [Mode==4]
  (junction 118) -> AOO_Charging [order 1] : [Mode==2]
  AOO_Pacing -> (junction 118) : after(A_Pulse_Width,msec){AdeltaT= AdeltaT+ uint16(A_Pulse_Width)}
  (junction 118) -> AAI [order 2] : [Mode==3]
  AOO_Charging -> AAI [order 2] : [Mode == 3 && ATR_CMP_DETECT == true]{AdeltaT = 0}
  AAI -> AOO_Charging : after(A_RefractoryPeriod, msec){AdeltaT = AdeltaT + A_RefractoryPeriod}
  DOO_Charging -> DOO_Pacing : after((60000/LRL) - A_Pulse_Width, msec)
  DOO_Pacing -> DOO_Charging1 : after(A_Pulse_Width, msec)
  DOO_Pacing1 -> DOO_Charging : after(V_Pulse_Width, msec)
  DOO_Charging1 -> DOO_Pacing1 : after((60000/uint16(LRL)) - uint16(V_Pulse_Width) + Fixed_AV_Delay, msec)
  data: Mode input; PACE_CHARGE_CTRL output; VENT_CMP_REF_PWM output; Z_ATR_CTRL output; PACING_REF_PWM output; ATR_CMP_REF_PWM output; Z_VENT_CTRL output; LRL input; URL input; A_Amplitude input; A_Pulse_Width input uint8; ATR_PACE_CTRL output; VENT_PACE_CTRL output; PACE_GND_CTRL output; ATR_GND_CTRL output; VENT_GND_CTRL output; FRONTEND_CTRL output; V_Amplitude input; V_Pulse_Width input uint8; A_RefractoryPeriod input uint16; RED_LED output; GREEN_LED output; BLUE_LED output; V_RefractoryPeriod input uint16; A_Sens input; V_Sens input; Rate_Smoothing input; PVARP input; ATR_CMP_DETECT input; VENT_CMP_DETECT input; AdeltaT local uint16; VdeltaT local uint16; Fixed_AV_Delay input; Max_Sensor_Rate input; Activity_Threshold input; Reaction_Time input; Response_Factor input; Recovery_Time input
